simulink model "Test_observer"  (R2019b)
settings: Solver=FixedStepAuto  StartTime=0.0  StopTime=5  FixedStep=20e-3  MaxStep=20e-3  MinStep=1e-3  RelTol=1e-1
values from neighbouring files (symbols this model uses):
  c_e = 0.0501    [model_parameters.m]
  c_m = 0.0514    [model_parameters.m]
  J_m = 71e-7    (= 7.1e-06)    [model_parameters.m]
  k_fric = 7.3e-3    (= 0.0073)    [model_parameters.m]
  k_i = 1.7e-3    (= 0.0017)    [model_parameters.m]
  k_p = 5.40    (= 5.4)    [model_parameters.m]
  L_a = 8.9e-3    (= 0.0089)    [model_parameters.m]
  R_a = 5.3361    [model_parameters.m]
undefined symbols (not defined in the file or in its folder): delta_dead_zone, tay
libraries: simulink x6, lib_robotinohardware x5
settings Model: EnablePacing=on  Creator=indorewala  LastModifiedBy=Олег
settings SolverCC: ZcThreshold=1e-1  MaxConsecutiveZCs=1e3  ZeroCrossAlgorithm=Adaptive
settings DataIOCC: LimitDataPoints=on  SaveFormat=Array  SignalLoggingSaveFormat=ModelDataLogs  ReturnWorkspaceOutputs=off
settings OptimizationCC: ExpressionDepthLimit=2147483647  InitFltsAndDblsToZero=on  LifeSpan=inf
settings DebuggingCC: UnderspecifiedInitializationDetection=Classic  MergeDetectMultiDrivingBlocksExec=none  SolverPrmCheckMsg=warning  FcnCallInpInsideContextMsg=warning  StateNameClashWarn=warning  SFUnexpectedBacktrackingDiag=warning  SFNoUnconditionalDefaultTransitionDiag=warning  SFExecutionAtInitializationDiag=none  ArithmeticOperatorsInVariantConditions=warning
settings HardwareCC: ProdBitPerPointer=32  ProdBitPerSizeT=32  ProdBitPerPtrDiffT=32  ProdLargestAtomicFloat=None  ProdIntDivRoundTo=Undefined  ProdEndianess=Unspecified  ProdWordSize=32  ProdHWDeviceType=32-bit Generic
settings ModelReferenceCC: PropagateSignalLabelsOutOfModel=off
settings SFSimCC: SimUseLocalCustomCode=off  CustomCodeUndefinedFunction=UseInterfaceOnly
settings RTWCC: RTWUseLocalCustomCode=off
settings CodeAppCC: StateflowObjectComments=on
settings GRTTargetCC: TargetLangStandard=C89/C90 (ANSI)  CombineOutputUpdateFcns=off  GRTInterface=on
settings ConfigComp: CovMetricSettings=dw  CovHtmlReporting=on  CovSaveCumulativeToWorkspaceVar=on  CovSaveSingleToWorkspaceVar=on  CovExternalEMLEnable=off

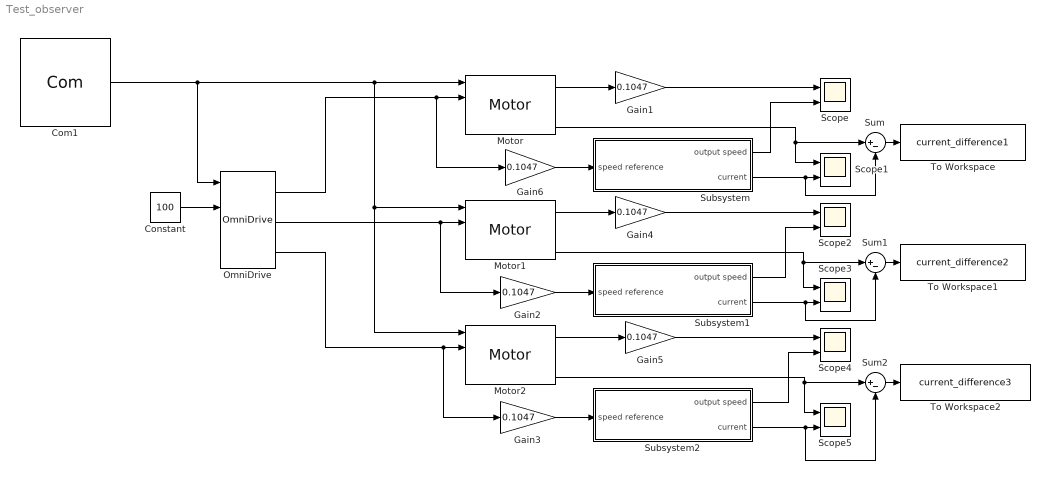
== system Test_observer ==
  Com1 : lib_robotinohardware/Com  ip='172.26.1.0'
  Constant : Constant  Value=100
  Gain{1..6} (6 alike) : Gain  Gain=0.1047
  Motor : lib_robotinohardware/Motor  num=0  kp=200  ki=10  kd=0
  Motor1 : lib_robotinohardware/Motor  num=1  kp=200  ki=10  kd=0
  Motor2 : lib_robotinohardware/Motor  num=2  kp=200  ki=10  kd=0
  OmniDrive : lib_robotinohardware/OmniDrive
  Scope{,1..5} (6 alike) : Scope  NumInputPorts=2
  Subsystem : Subsystem
  Subsystem1 : Subsystem
  Subsystem2 : Subsystem
  Sum : Sum  Inputs=|+-
  Sum1 : Sum  Inputs=|+-
  Sum2 : Sum  Inputs=|+-
  To Workspace : ToWorkspace  VariableName=current_difference1  SaveFormat=Timeseries  SampleTime=-1
  To Workspace1 : ToWorkspace  VariableName=current_difference2  SaveFormat=Timeseries  SampleTime=-1
  To Workspace2 : ToWorkspace  VariableName=current_difference3  SaveFormat=Timeseries  SampleTime=-1
  wires:
  Com1/1 -> OmniDrive/1, Motor/1, Motor2/1, Motor1/1
  Motor/1 -> Gain1/1
  OmniDrive/1 -> Gain6/1, Motor/2
  OmniDrive/2 -> Gain2/1, Motor1/2
  OmniDrive/3 -> Gain3/1, Motor2/2
  Gain1/1 -> Scope/1
  Motor/3 -> Sum/1, Scope1/1
  Gain6/1 -> Subsystem/1(speed reference)
  Subsystem/1(output speed) -> Scope/2
  Subsystem/2(current) -> Sum/2, Scope1/2
  Gain2/1 -> Subsystem1/1(speed reference)
  Gain3/1 -> Subsystem2/1(speed reference)
  Motor1/1 -> Gain4/1
  Gain4/1 -> Scope2/1
  Subsystem1/1(output speed) -> Scope2/2
  Motor1/3 -> Sum1/1, Scope3/1
  Subsystem2/1(output speed) -> Scope4/2
  Motor2/1 -> Gain5/1
  Gain5/1 -> Scope4/1
  Motor2/3 -> Sum2/1, Scope5/1
  Sum/1 -> To Workspace/1
  Sum1/1 -> To Workspace1/1
  Subsystem1/2(current) -> Sum1/2, Scope3/2
  Subsystem2/2(current) -> Sum2/2, Scope5/2
  Sum2/1 -> To Workspace2/1
  Constant/1 -> OmniDrive/2

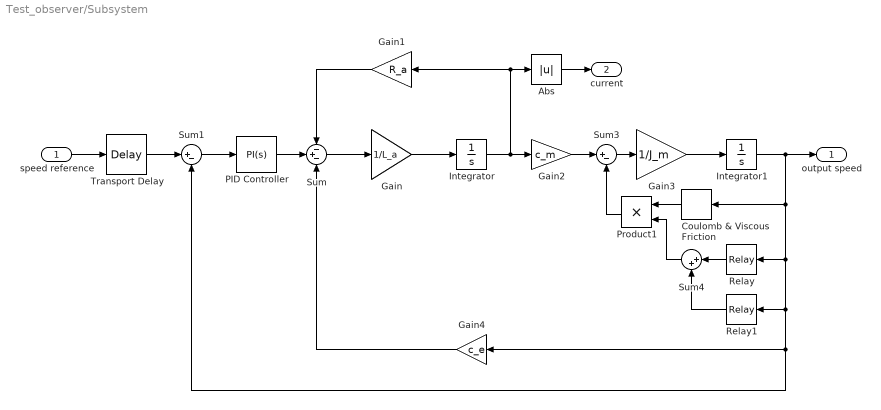
== system Test_observer/Subsystem ==
  speed reference : Inport
  Abs : Abs
  Coulomb & Viscous Friction : simulink/Discontinuities/Coulomb & Viscous Friction  offset=M_dist  gain=k_fric
      settings: SourceProductName=Simulink
  Gain : Gain  Gain=1/L_a
  Gain1 : Gain  Gain=R_a
  Gain2 : Gain  Gain=c_m
  Gain3 : Gain  Gain=1/J_m
  Gain4 : Gain  Gain=c_e
  Integrator : Integrator
  Integrator1 : Integrator
  PID Controller : simulink/Continuous/PID Controller  Controller=PI  Form=Parallel  TimeDomain=Continuous-time  SampleTime=-1  IntegratorMethod=Forward Euler  FilterMethod=Forward Euler  ControllerParametersSource=internal  P=k_p  I=k_i  D=0  UseFilter=on  N=100  TunerSelectOption=Transfer Function Based (PID Tuner App)  InitialConditionSource=internal  InitialConditionForIntegrator=0  InitialConditionForFilter=0  DifferentiatorICPrevScaledInput=0  ExternalReset=none  TrackingMode=off  Kt=1  LimitOutput=off  UpperSaturationLimit=inf  LowerSaturationLimit=-inf  LinearizeAsGain=on  AntiWindupMode=none  Kb=1  POutMin=[]  POutMax=[]  IOutMin=[]  IOutMax=[]  DOutMin=[]  DOutMax=[]  NOutMin=[]  NOutMax=[]  SumOutMin=[]  SumOutMax=[]  SaturationOutMin=[]  SaturationOutMax=[]  PParamMin=[]  PParamMax=[]  IParamMin=[]  IParamMax=[]  DParamMin=[]  DParamMax=[]  NParamMin=[]  NParamMax=[]  KbParamMin=[]  KbParamMax=[]  KtParamMin=[]  KtParamMax=[]  KbOutMin=[]  KbOutMax=[]  KtOutMin=[]  KtOutMax=[]  IntegratorOutMin=[]  IntegratorOutMax=[]  FilterOutMin=[]  FilterOutMax=[]  SumI1OutMin=[]  SumI1OutMax=[]  SumI2OutMin=[]  SumI2OutMax=[]  SumI3OutMin=[]  SumI3OutMax=[]  SumI4OutMin=[]  SumI4OutMax=[]  SumDOutMin=[]  SumDOutMax=[]  DifferentiatorOutMin=[]  DifferentiatorOutMax=[]  FilterDiffOutCoefMin=[]  FilterDiffOutCoefMax=[]  ReciprocalOutMin=[]  ReciprocalOutMax=[]  SumDenOutMin=[]  SumDenOutMax=[]  SumNumOutMin=[]  SumNumOutMax=[]  DivideOutMin=[]  DivideOutMax=[]  IntegratorContinuousStateAttributes=''  IntegratorStateMustResolveToSignalObject=off  IntegratorRTWStateStorageClass=Auto  FilterContinuousStateAttributes=''  FilterStateMustResolveToSignalObject=off  FilterRTWStateStorageClass=Auto  ParallelPVariant=InternalParameters  IdealPVariant=Disabled  IVariant=InternalParameters  DVariant=Disabled  IntegratorVariant=Continuous  SatVariant=Disabled  AWVariant=Passthrough  PCopyVariant=Disabled  TRVariant=Disabled  FdbkBlocksVariant=Forward  IdealPFdbkVariant=Disabled  SatFdbkVariant=Disabled  DerivativeFilterVariant=Disabled  NVariant=Disabled  NCopyVariant=Disabled_SignalSpec  FilterICVariant=Disabled  IntegratorICVariant=InternalICs  ExternalResetVariant=Disabled  TRSumVariant=Passthrough  SumFdbkVariant=Disabled  SumVariant=Sum_PI
  Product1 : Product
  Relay : Relay  OnSwitchValue=-delta_dead_zone  OffSwitchValue=-delta_dead_zone  OnOutputValue=0  OffOutputValue=1
  Relay1 : Relay  OnSwitchValue=delta_dead_zone  OffSwitchValue=delta_dead_zone
  Sum : Sum  Inputs=-+-
  Sum1 : Sum  Inputs=|+-
  Sum3 : Sum  Inputs=|+-
  Sum4 : Sum  Inputs=|++
  Transport Delay : TransportDelay  DelayTime=tay
  output speed : Outport
  current : Outport  Port=2
  wires:
  Product1/1 -> Sum3/2
  Sum3/1 -> Gain3/1
  Gain3/1 -> Integrator1/1
  Transport Delay/1 -> Sum1/1
  Integrator1/1 -> output speed/1, Coulomb & Viscous Friction/1, Relay/1, Relay1/1, Gain4/1, Sum1/2
  Sum4/1 -> Product1/2
  Relay1/1 -> Sum4/2
  Integrator/1 -> Gain2/1, Abs/1, Gain1/1
  PID Controller/1 -> Sum/2
  Relay/1 -> Sum4/1
  Gain1/1 -> Sum/1
  speed reference/1 -> Transport Delay/1
  Coulomb & Viscous Friction/1 -> Product1/1
  Sum1/1 -> PID Controller/1
  Gain2/1 -> Sum3/1
  Gain4/1 -> Sum/3
  Sum/1 -> Gain/1
  Abs/1 -> current/1
  Gain/1 -> Integrator/1

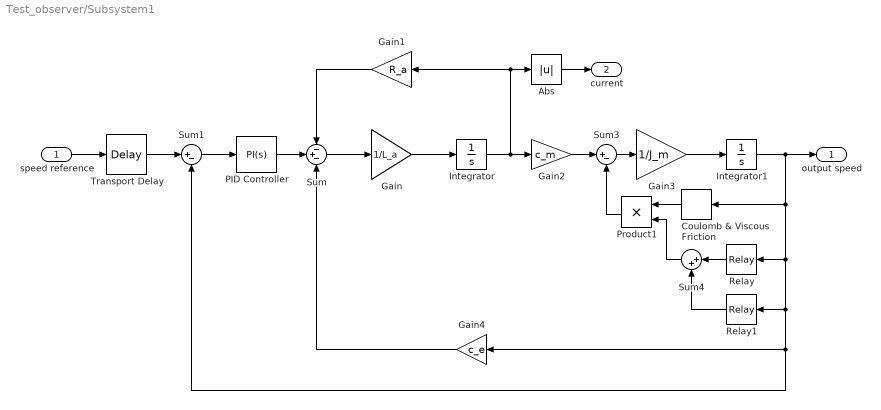
== system Test_observer/Subsystem1 ==
  speed reference : Inport
  Abs : Abs
  Coulomb & Viscous Friction : simulink/Discontinuities/Coulomb & Viscous Friction  offset=M_dist  gain=k_fric
      settings: SourceProductName=Simulink
  Gain : Gain  Gain=1/L_a
  Gain1 : Gain  Gain=R_a
  Gain2 : Gain  Gain=c_m
  Gain3 : Gain  Gain=1/J_m
  Gain4 : Gain  Gain=c_e
  Integrator : Integrator
  Integrator1 : Integrator
  PID Controller : simulink/Continuous/PID Controller  Controller=PI  Form=Parallel  TimeDomain=Continuous-time  SampleTime=-1  IntegratorMethod=Forward Euler  FilterMethod=Forward Euler  ControllerParametersSource=internal  P=k_p  I=k_i  D=0  UseFilter=on  N=100  TunerSelectOption=Transfer Function Based (PID Tuner App)  InitialConditionSource=internal  InitialConditionForIntegrator=0  InitialConditionForFilter=0  DifferentiatorICPrevScaledInput=0  ExternalReset=none  TrackingMode=off  Kt=1  LimitOutput=off  UpperSaturationLimit=inf  LowerSaturationLimit=-inf  LinearizeAsGain=on  AntiWindupMode=none  Kb=1  POutMin=[]  POutMax=[]  IOutMin=[]  IOutMax=[]  DOutMin=[]  DOutMax=[]  NOutMin=[]  NOutMax=[]  SumOutMin=[]  SumOutMax=[]  SaturationOutMin=[]  SaturationOutMax=[]  PParamMin=[]  PParamMax=[]  IParamMin=[]  IParamMax=[]  DParamMin=[]  DParamMax=[]  NParamMin=[]  NParamMax=[]  KbParamMin=[]  KbParamMax=[]  KtParamMin=[]  KtParamMax=[]  KbOutMin=[]  KbOutMax=[]  KtOutMin=[]  KtOutMax=[]  IntegratorOutMin=[]  IntegratorOutMax=[]  FilterOutMin=[]  FilterOutMax=[]  SumI1OutMin=[]  SumI1OutMax=[]  SumI2OutMin=[]  SumI2OutMax=[]  SumI3OutMin=[]  SumI3OutMax=[]  SumI4OutMin=[]  SumI4OutMax=[]  SumDOutMin=[]  SumDOutMax=[]  DifferentiatorOutMin=[]  DifferentiatorOutMax=[]  FilterDiffOutCoefMin=[]  FilterDiffOutCoefMax=[]  ReciprocalOutMin=[]  ReciprocalOutMax=[]  SumDenOutMin=[]  SumDenOutMax=[]  SumNumOutMin=[]  SumNumOutMax=[]  DivideOutMin=[]  DivideOutMax=[]  IntegratorContinuousStateAttributes=''  IntegratorStateMustResolveToSignalObject=off  IntegratorRTWStateStorageClass=Auto  FilterContinuousStateAttributes=''  FilterStateMustResolveToSignalObject=off  FilterRTWStateStorageClass=Auto  ParallelPVariant=InternalParameters  IdealPVariant=Disabled  IVariant=InternalParameters  DVariant=Disabled  IntegratorVariant=Continuous  SatVariant=Disabled  AWVariant=Passthrough  PCopyVariant=Disabled  TRVariant=Disabled  FdbkBlocksVariant=Forward  IdealPFdbkVariant=Disabled  SatFdbkVariant=Disabled  DerivativeFilterVariant=Disabled  NVariant=Disabled  NCopyVariant=Disabled_SignalSpec  FilterICVariant=Disabled  IntegratorICVariant=InternalICs  ExternalResetVariant=Disabled  TRSumVariant=Passthrough  SumFdbkVariant=Disabled  SumVariant=Sum_PI
  Product1 : Product
  Relay : Relay  OnSwitchValue=-delta_dead_zone  OffSwitchValue=-delta_dead_zone  OnOutputValue=0  OffOutputValue=1
  Relay1 : Relay  OnSwitchValue=delta_dead_zone  OffSwitchValue=delta_dead_zone
  Sum : Sum  Inputs=-+-
  Sum1 : Sum  Inputs=|+-
  Sum3 : Sum  Inputs=|+-
  Sum4 : Sum  Inputs=|++
  Transport Delay : TransportDelay  DelayTime=tay
  output speed : Outport
  current : Outport  Port=2
  wires:
  Product1/1 -> Sum3/2
  Sum3/1 -> Gain3/1
  Gain3/1 -> Integrator1/1
  Transport Delay/1 -> Sum1/1
  Integrator1/1 -> output speed/1, Coulomb & Viscous Friction/1, Relay/1, Relay1/1, Gain4/1, Sum1/2
  Sum4/1 -> Product1/2
  Relay1/1 -> Sum4/2
  Integrator/1 -> Gain2/1, Abs/1, Gain1/1
  PID Controller/1 -> Sum/2
  Relay/1 -> Sum4/1
  Gain1/1 -> Sum/1
  speed reference/1 -> Transport Delay/1
  Coulomb & Viscous Friction/1 -> Product1/1
  Sum1/1 -> PID Controller/1
  Gain2/1 -> Sum3/1
  Gain4/1 -> Sum/3
  Sum/1 -> Gain/1
  Abs/1 -> current/1
  Gain/1 -> Integrator/1

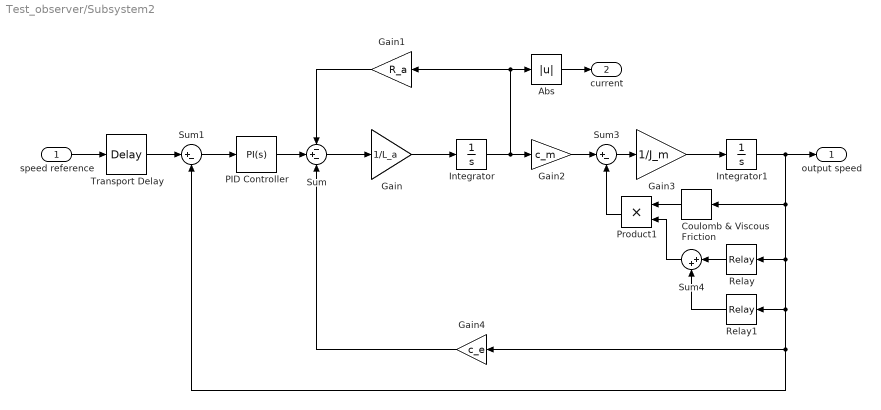
== system Test_observer/Subsystem2 ==
  speed reference : Inport
  Abs : Abs
  Coulomb & Viscous Friction : simulink/Discontinuities/Coulomb & Viscous Friction  offset=M_dist  gain=k_fric
      settings: SourceProductName=Simulink
  Gain : Gain  Gain=1/L_a
  Gain1 : Gain  Gain=R_a
  Gain2 : Gain  Gain=c_m
  Gain3 : Gain  Gain=1/J_m
  Gain4 : Gain  Gain=c_e
  Integrator : Integrator
  Integrator1 : Integrator
  PID Controller : simulink/Continuous/PID Controller  Controller=PI  Form=Parallel  TimeDomain=Continuous-time  SampleTime=-1  IntegratorMethod=Forward Euler  FilterMethod=Forward Euler  ControllerParametersSource=internal  P=k_p  I=k_i  D=0  UseFilter=on  N=100  TunerSelectOption=Transfer Function Based (PID Tuner App)  InitialConditionSource=internal  InitialConditionForIntegrator=0  InitialConditionForFilter=0  DifferentiatorICPrevScaledInput=0  ExternalReset=none  TrackingMode=off  Kt=1  LimitOutput=off  UpperSaturationLimit=inf  LowerSaturationLimit=-inf  LinearizeAsGain=on  AntiWindupMode=none  Kb=1  POutMin=[]  POutMax=[]  IOutMin=[]  IOutMax=[]  DOutMin=[]  DOutMax=[]  NOutMin=[]  NOutMax=[]  SumOutMin=[]  SumOutMax=[]  SaturationOutMin=[]  SaturationOutMax=[]  PParamMin=[]  PParamMax=[]  IParamMin=[]  IParamMax=[]  DParamMin=[]  DParamMax=[]  NParamMin=[]  NParamMax=[]  KbParamMin=[]  KbParamMax=[]  KtParamMin=[]  KtParamMax=[]  KbOutMin=[]  KbOutMax=[]  KtOutMin=[]  KtOutMax=[]  IntegratorOutMin=[]  IntegratorOutMax=[]  FilterOutMin=[]  FilterOutMax=[]  SumI1OutMin=[]  SumI1OutMax=[]  SumI2OutMin=[]  SumI2OutMax=[]  SumI3OutMin=[]  SumI3OutMax=[]  SumI4OutMin=[]  SumI4OutMax=[]  SumDOutMin=[]  SumDOutMax=[]  DifferentiatorOutMin=[]  DifferentiatorOutMax=[]  FilterDiffOutCoefMin=[]  FilterDiffOutCoefMax=[]  ReciprocalOutMin=[]  ReciprocalOutMax=[]  SumDenOutMin=[]  SumDenOutMax=[]  SumNumOutMin=[]  SumNumOutMax=[]  DivideOutMin=[]  DivideOutMax=[]  IntegratorContinuousStateAttributes=''  IntegratorStateMustResolveToSignalObject=off  IntegratorRTWStateStorageClass=Auto  FilterContinuousStateAttributes=''  FilterStateMustResolveToSignalObject=off  FilterRTWStateStorageClass=Auto  ParallelPVariant=InternalParameters  IdealPVariant=Disabled  IVariant=InternalParameters  DVariant=Disabled  IntegratorVariant=Continuous  SatVariant=Disabled  AWVariant=Passthrough  PCopyVariant=Disabled  TRVariant=Disabled  FdbkBlocksVariant=Forward  IdealPFdbkVariant=Disabled  SatFdbkVariant=Disabled  DerivativeFilterVariant=Disabled  NVariant=Disabled  NCopyVariant=Disabled_SignalSpec  FilterICVariant=Disabled  IntegratorICVariant=InternalICs  ExternalResetVariant=Disabled  TRSumVariant=Passthrough  SumFdbkVariant=Disabled  SumVariant=Sum_PI
  Product1 : Product
  Relay : Relay  OnSwitchValue=-delta_dead_zone  OffSwitchValue=-delta_dead_zone  OnOutputValue=0  OffOutputValue=1
  Relay1 : Relay  OnSwitchValue=delta_dead_zone  OffSwitchValue=delta_dead_zone
  Sum : Sum  Inputs=-+-
  Sum1 : Sum  Inputs=|+-
  Sum3 : Sum  Inputs=|+-
  Sum4 : Sum  Inputs=|++
  Transport Delay : TransportDelay  DelayTime=tay
  output speed : Outport
  current : Outport  Port=2
  wires:
  Product1/1 -> Sum3/2
  Sum3/1 -> Gain3/1
  Gain3/1 -> Integrator1/1
  Transport Delay/1 -> Sum1/1
  Integrator1/1 -> output speed/1, Coulomb & Viscous Friction/1, Relay/1, Relay1/1, Gain4/1, Sum1/2
  Sum4/1 -> Product1/2
  Relay1/1 -> Sum4/2
  Integrator/1 -> Gain2/1, Abs/1, Gain1/1
  PID Controller/1 -> Sum/2
  Relay/1 -> Sum4/1
  Gain1/1 -> Sum/1
  speed reference/1 -> Transport Delay/1
  Coulomb & Viscous Friction/1 -> Product1/1
  Sum1/1 -> PID Controller/1
  Gain2/1 -> Sum3/1
  Gain4/1 -> Sum/3
  Sum/1 -> Gain/1
  Abs/1 -> current/1
  Gain/1 -> Integrator/1
